simulink model "tx2"  (R2022a)
settings: Solver=FixedStepDiscrete  StartTime=0.0  StopTime=3.1e6  FixedStep=1  RelTol=1e-3
undefined symbols (not defined in the file or in its folder): rom_bf1, rom_bf2, rom_bf3, rom_bf4, rom_bf5, rom_bf6, rom_bf7, rom_bf8, rom_pilot_tt
libraries: hdlsllib x809, whdlutilities x460, whdlmod x104, whdledac x26, simulink x3
(part 8 of 27)

== system tx2/Subsystem6/mapping_process_L1 ==
  data_in : Inport  OutDataTypeStr=boolean
  mapping_ctrl : Inport  Port=2  OutDataTypeStr=Bus: samplecontrol
  Constant : Constant  Value=sqrt(2)/2  OutDataTypeStr=fixdt(1,16,14)
  Constant1 : Constant  Value=-sqrt(2)/2  OutDataTypeStr=fixdt(1,16,14)
  Constant2 : Constant  Value=0  OutDataTypeStr=uint8
  Constant3 : Constant  Value=0  OutDataTypeStr=fixdt(1,16,14)
  Delay : Delay  DelayLength=1  InitialCondition=0  ShowEnablePort=on
      settings: InputPortMap=u0,e6
  Delay{1,5..8,10..12} (8 alike) : Delay  DelayLength=1  InitialCondition=0
  Delay{3..4,9,13} (4 alike) : Delay  InitialCondition=0
  Delay2 : Delay  DelayLength=1  InitialCondition=0  ShowEnablePort=on
      settings: InputPortMap=u0,e6
  Demux : Demux  Outputs=2
  Logical Operator : Logic  Operator=OR  AllPortsSameDT=off  OutDataTypeStr=boolean
  Logical Operator1 : Logic  AllPortsSameDT=off  OutDataTypeStr=boolean
  Logical Operator13 : Logic  Operator=NOT  AllPortsSameDT=off  OutDataTypeStr=boolean
  Real-Imag to Complex : RealImagToComplex
  Real-Imag to Complex1 : RealImagToComplex
  Sample Control Bus Creator : whdlutilities/Sample Control Bus Creator
      settings: SourceProductBaseCode=LH
  Sample Control Bus Creator1 : whdlutilities/Sample Control Bus Creator
      settings: SourceProductBaseCode=LH
  Sample Control Bus Selector : whdlutilities/Sample Control Bus Selector  OutputSignals=start,end,valid
      settings: SourceProductBaseCode=LH
  Switch{,1..3} (4 alike) : Switch  Criteria=u2 ~= 0  SaturateOnIntegerOverflow=off  InputSameDT=off
  "divide6 " : hdlsllib/Sources/HDL Counter  CountType=Count limited  CountInit=1  CountStep=1  CountMax=12  CountFromType=Initial value  CountFrom=1  CountResetPort=on  CountLoadPort=off  CountEnbPort=on  CountDirPort=off  CountHitOutputPort=on  CountDataType=Unsigned  CountWordLen=8  CountFracLen=0  CountSampTime=1
  divide6 1 : hdlsllib/Sources/HDL Counter  CountType=Count limited  CountInit=1  CountStep=1  CountMax=6*12  CountFromType=Initial value  CountFrom=1  CountResetPort=on  CountLoadPort=off  CountEnbPort=on  CountDirPort=off  CountHitOutputPort=off  CountDataType=Unsigned  CountWordLen=8  CountFracLen=0  CountSampTime=1
  data_out : Outport  VectorParamsAs1DForOutWhenUnconnected=off
      settings: SignalType=complex
  ctrl_mapping : Outport  Port=2  OutDataTypeStr=Bus: samplecontrol  VectorParamsAs1DForOutWhenUnconnected=off
  RB_ctrl : Outport  Port=3  OutDataTypeStr=Bus: samplecontrol  VectorParamsAs1DForOutWhenUnconnected=off
  RB_id : Outport  Port=4  OutDataTypeStr=uint8  VectorParamsAs1DForOutWhenUnconnected=off
  wires:
  Switch1/1 -> Real-Imag to Complex/2
  Switch/1 -> Real-Imag to Complex/1
  Delay/1 -> Demux/1
  Demux/1 -> Switch/2
  Demux/2 -> Switch1/2
  Real-Imag to Complex/1 -> Delay2/1
  Delay2/1 -> Delay6/1
  Delay3/1 -> Delay5/1
  Delay1/1 -> Delay2/2, Delay13/1
  mapping_ctrl/1 -> Sample Control Bus Selector/1
  "divide6 "/2 -> divide6 1/2, Delay11/1, Delay10/1  "count6"
  Logical Operator13/1 -> divide6 1/1, "divide6 "/1
  Sample Control Bus Selector/1 -> Delay9/1, Sample Control Bus Creator/1  "<start>"
  Sample Control Bus Selector/2 -> Sample Control Bus Creator/2  "<end>"
  Sample Control Bus Selector/3 -> Sample Control Bus Creator/3, Delay4/1, Delay1/1, Delay/2  "<valid>"
  Sample Control Bus Creator/1 -> Delay3/1
  divide6 1/1 -> Switch2/1  "RB_id"
  Delay4/1 -> Logical Operator13/1, "divide6 "/2, Delay12/1, Switch2/2, Logical Operator1/1
  Switch2/1 -> Delay7/1
  Constant2/1 -> Switch2/3
  Delay6/1 -> Switch3/1
  Logical Operator/1 -> Logical Operator1/2
  Delay9/1 -> Logical Operator/2
  Delay10/1 -> Logical Operator/1
  Logical Operator1/1 -> Delay8/1
  Delay8/1 -> Sample Control Bus Creator1/1
  Delay11/1 -> Sample Control Bus Creator1/2
  Delay12/1 -> Sample Control Bus Creator1/3
  Delay5/1 -> ctrl_mapping/1
  Delay7/1 -> RB_id/1
  Sample Control Bus Creator1/1 -> RB_ctrl/1
  data_in/1 -> Delay/1  "data_with_CP"
  Switch3/1 -> data_out/1
  Constant3/1 -> Real-Imag to Complex1/2, Real-Imag to Complex1/1
  Real-Imag to Complex1/1 -> Switch3/3
  Delay13/1 -> Switch3/2
  Constant/1 -> Switch1/3, Switch/3
  Constant1/1 -> Switch/1, Switch1/1

== system tx2/Subsystem7/BF ==
  layer_data_in1 : Inport
  BF_data_ctrl : Inport  Port=2  OutDataTypeStr=Bus: samplecontrol
  RB_id : Inport  Port=3  OutDataTypeStr=uint8
  RB_id_ctrl : Inport  Port=4  OutDataTypeStr=Bus: samplecontrol
  Delay{,3..8,10} (8 alike) : Delay  DelayLength=1  InitialCondition=0
  Delay1 : Delay  InitialCondition=0
  Delay2 : Delay  DelayLength=3  InitialCondition=0
  Delay9 : Delay  InitialCondition=0
  Logical Operator : Logic  Operator=NOT  AllPortsSameDT=off  OutDataTypeStr=boolean
  Mux : Mux  Inputs=8
  Product{,1..7} (8 alike) : Product  OutDataTypeStr=fixdt(1,16,14)  LockScale=on
  Sample Control Bus Selector : whdlutilities/Sample Control Bus Selector  OutputSignals=start,end,valid
      settings: SourceProductBaseCode=LH
  Sample Control Bus Selector1 : whdlutilities/Sample Control Bus Selector  OutputSignals=start,end,valid
      settings: SourceProductBaseCode=LH
  address controller : hdlsllib/Sources/HDL Counter  CountType=Count limited  CountInit=0  CountStep=1  CountMax=7  CountFromType=Initial value  CountFrom=0  CountResetPort=on  CountLoadPort=off  CountEnbPort=on  CountDirPort=off  CountHitOutputPort=off  CountDataType=Unsigned  CountWordLen=8  CountFracLen=0  CountSampTime=1
  rom_bf1 : Subsystem
  rom_bf2 : Subsystem
  rom_bf3 : Subsystem
  rom_bf4 : Subsystem
  rom_bf5 : Subsystem
  rom_bf6 : Subsystem
  rom_bf7 : Subsystem
  rom_bf8 : Subsystem
  process_bf : Outport  PortDimensions=8  VectorParamsAs1DForOutWhenUnconnected=off
  BF_ctrl : Outport  Port=2  OutDataTypeStr=Bus: samplecontrol  VectorParamsAs1DForOutWhenUnconnected=off
  RB_n_bf : Outport  Port=3  VectorParamsAs1DForOutWhenUnconnected=off
  wires:
  Delay1/1 -> Product7/1, Product6/1, Product5/1, Product4/1, Product3/1, Product2/1, Product1/1, Product/1
  rom_bf1/1(data_out) -> Product/2
  Product/1 -> Delay/1
  Delay2/1 -> BF_ctrl/1  "BF_ctrl"
  address controller/1 -> rom_bf7/1(address), rom_bf8/1(address), rom_bf6/1(address), rom_bf5/1(address), rom_bf4/1(address), rom_bf3/1(address), rom_bf2/1(address), rom_bf1/1(address)
  Delay9/1 -> RB_n_bf/1  "RB_ID"
  RB_id_ctrl/1 -> Sample Control Bus Selector1/1
  BF_data_ctrl/1 -> Delay2/1, Sample Control Bus Selector/1
  Sample Control Bus Selector1/2 -> address controller/2  "<end>"
  RB_id/1 -> Delay9/1
  layer_data_in1/1 -> Delay1/1
  Sample Control Bus Selector/3 -> rom_bf2/2(read_en), rom_bf1/2(read_en), rom_bf3/2(read_en), rom_bf4/2(read_en), rom_bf5/2(read_en), rom_bf6/2(read_en), rom_bf7/2(read_en), rom_bf8/2(read_en)  "<valid>"
  Product1/1 -> Delay3/1
  Product2/1 -> Delay4/1
  Product4/1 -> Delay6/1
  Product3/1 -> Delay5/1
  Product5/1 -> Delay7/1
  Product6/1 -> Delay8/1
  rom_bf2/1(data_out) -> Product1/2
  rom_bf3/1(data_out) -> Product2/2
  rom_bf4/1(data_out) -> Product3/2
  rom_bf5/1(data_out) -> Product4/2
  rom_bf6/1(data_out) -> Product5/2
  Product7/1 -> Delay10/1
  rom_bf7/1(data_out) -> Product6/2
  rom_bf8/1(data_out) -> Product7/2
  Delay3/1 -> Mux/2
  Delay4/1 -> Mux/3
  Delay5/1 -> Mux/4
  Delay10/1 -> Mux/8
  Delay8/1 -> Mux/7
  Delay7/1 -> Mux/6
  Delay6/1 -> Mux/5
  Delay/1 -> Mux/1
  Mux/1 -> process_bf/1
  Sample Control Bus Selector1/3 -> Logical Operator/1  "<valid>"
  Logical Operator/1 -> address controller/1

== system tx2/Subsystem7/OFDM_process1 ==
  process_bf : Inport
  BF_ctrl : Inport  Port=2
  Demux : Demux  Outputs=8
  OFDM_process1_bf1 : Subsystem
  OFDM_process1_bf2 : Subsystem
  OFDM_process1_bf3 : Subsystem
  OFDM_process1_bf4 : Subsystem
  OFDM_process1_bf5 : Subsystem
  OFDM_process1_bf6 : Subsystem
  OFDM_process1_bf7 : Subsystem
  OFDM_process1_bf8 : Subsystem
  OFDM_bf1 : Outport
  OFDM_ctrl_bf1 : Outport  Port=2
  OFDM_bf2 : Outport  Port=3
  OFDM_ctrl_bf2 : Outport  Port=4
  OFDM_bf3 : Outport  Port=5
  OFDM_ctrl_bf3 : Outport  Port=6
  OFDM_bf4 : Outport  Port=7
  OFDM_ctrl_bf4 : Outport  Port=8
  OFDM_bf5 : Outport  Port=9
  OFDM_ctrl_bf5 : Outport  Port=10
  OFDM_bf6 : Outport  Port=11
  OFDM_ctrl_bf6 : Outport  Port=12
  OFDM_bf7 : Outport  Port=13
  OFDM_ctrl_bf7 : Outport  Port=14
  OFDM_bf8 : Outport  Port=15
  OFDM_ctrl_bf8 : Outport  Port=16
  wires:
  Demux/3 -> OFDM_process1_bf3/1(data)  "bf3"
  Demux/1 -> OFDM_process1_bf1/1(data)  "bf1"
  BF_ctrl/1 -> OFDM_process1_bf7/2(BF_ctrl), OFDM_process1_bf8/2(BF_ctrl), OFDM_process1_bf6/2(BF_ctrl), OFDM_process1_bf5/2(BF_ctrl), OFDM_process1_bf4/2(BF_ctrl), OFDM_process1_bf3/2(BF_ctrl), OFDM_process1_bf2/2(BF_ctrl), OFDM_process1_bf1/2(BF_ctrl)
  Demux/5 -> OFDM_process1_bf5/1(data)  "bf5"
  OFDM_process1_bf1/2(OFDM_ctrl_process) -> OFDM_ctrl_bf1/1
  OFDM_process1_bf2/2(OFDM_ctrl_process) -> OFDM_ctrl_bf2/1
  Demux/2 -> OFDM_process1_bf2/1(data)  "bf2"
  Demux/4 -> OFDM_process1_bf4/1(data)  "bf4"
  OFDM_process1_bf8/2(OFDM_ctrl_process) -> OFDM_ctrl_bf8/1
  Demux/8 -> OFDM_process1_bf8/1(data)  "bf8"
  Demux/7 -> OFDM_process1_bf7/1(data)  "bf7"
  Demux/6 -> OFDM_process1_bf6/1(data)  "bf6"
  OFDM_process1_bf7/2(OFDM_ctrl_process) -> OFDM_ctrl_bf7/1
  OFDM_process1_bf6/1(OFDM_process) -> OFDM_bf6/1
  OFDM_process1_bf3/1(OFDM_process) -> OFDM_bf3/1
  OFDM_process1_bf6/2(OFDM_ctrl_process) -> OFDM_ctrl_bf6/1
  OFDM_process1_bf5/1(OFDM_process) -> OFDM_bf5/1
  OFDM_process1_bf1/1(OFDM_process) -> OFDM_bf1/1
  OFDM_process1_bf8/1(OFDM_process) -> OFDM_bf8/1
  OFDM_process1_bf4/2(OFDM_ctrl_process) -> OFDM_ctrl_bf4/1
  OFDM_process1_bf3/2(OFDM_ctrl_process) -> OFDM_ctrl_bf3/1
  OFDM_process1_bf5/2(OFDM_ctrl_process) -> OFDM_ctrl_bf5/1
  process_bf/1 -> Demux/1
  OFDM_process1_bf7/1(OFDM_process) -> OFDM_bf7/1
  OFDM_process1_bf4/1(OFDM_process) -> OFDM_bf4/1
  OFDM_process1_bf2/1(OFDM_process) -> OFDM_bf2/1

== system tx2/Subsystem7/bit_level ==
  note: 此时的输出本身具有一位延迟
  process_data : Inport
  process_valid : Inport  Port=2  OutDataTypeStr=Bus: samplecontrol
  Compare To Constant1 : hdlsllib/Logic and Bit Operations/Compare To Constant  relop=<  const=385  OutDataTypeStr=boolean
      settings: SourceProductBaseCode=SL
  Compare To Constant2 : hdlsllib/Logic and Bit Operations/Compare To Constant  relop===  const=1584+192  OutDataTypeStr=boolean
      settings: SourceProductBaseCode=SL
  Compare To Constant3 : hdlsllib/Logic and Bit Operations/Compare To Constant  relop=>  const=576  OutDataTypeStr=boolean
      settings: SourceProductBaseCode=SL
  Compare To Constant4 : hdlsllib/Logic and Bit Operations/Compare To Constant  relop=<=  const=1584+192  OutDataTypeStr=boolean
      settings: SourceProductBaseCode=SL
  Compare To Constant5 : hdlsllib/Logic and Bit Operations/Compare To Constant  relop=>=  const=792+1  OutDataTypeStr=boolean
      settings: SourceProductBaseCode=SL
  Compare To Constant6 : hdlsllib/Logic and Bit Operations/Compare To Constant  relop=<=  const=1584  OutDataTypeStr=boolean
      settings: SourceProductBaseCode=SL
  Constant : Constant  OutDataTypeStr=boolean
  Constant1 : Constant  Value=72  OutDataTypeStr=uint16
  Constant2 : Constant  Value=0  OutDataTypeStr=boolean
  Constant3 : Constant  Value=0  OutDataTypeStr=fixdt(0,12,0)
  Data Type Conversion1 : DataTypeConversion  OutDataTypeStr=fixdt(0,1,0)  SaturateOnIntegerOverflow=off  RndMeth=Floor
  Data Type Conversion2 : DataTypeConversion  OutDataTypeStr=boolean  SaturateOnIntegerOverflow=off  RndMeth=Floor
  Data Type Conversion3 : DataTypeConversion  OutDataTypeStr=boolean  SaturateOnIntegerOverflow=off  RndMeth=Floor
  Delay1 : Delay  DelayLength=1  InitialCondition=0
  Delay2 : Delay  DelayLength=1  InitialCondition=0
  HDL Counter1 : hdlsllib/Sources/HDL Counter  CountType=Count limited  CountInit=1  CountStep=1  CountMax=1584  CountFromType=Initial value  CountFrom=1  CountResetPort=on  CountLoadPort=off  CountEnbPort=on  CountDirPort=off  CountHitOutputPort=off  CountDataType=Unsigned  CountWordLen=12  CountFracLen=0  CountSampTime=1
  HDL Counter2 : hdlsllib/Sources/HDL Counter  CountType=Count limited  CountInit=1  CountStep=1  CountMax=792  CountFromType=Initial value  CountFrom=1  CountResetPort=on  CountLoadPort=off  CountEnbPort=on  CountDirPort=off  CountHitOutputPort=off  CountDataType=Unsigned  CountWordLen=12  CountFracLen=0  CountSampTime=1
  HDL Counter4 : hdlsllib/Sources/HDL Counter  CountType=Count limited  CountInit=1  CountStep=1  CountMax=4096-1  CountFromType=Initial value  CountFrom=1  CountResetPort=on  CountLoadPort=off  CountEnbPort=on  CountDirPort=off  CountHitOutputPort=off  CountDataType=Unsigned  CountWordLen=12  CountFracLen=0  CountSampTime=1
  HDL Counter5 : hdlsllib/Sources/HDL Counter  CountType=Count limited  CountInit=0  CountStep=1  CountMax=1  CountFromType=Initial value  CountFrom=0  CountResetPort=on  CountLoadPort=off  CountEnbPort=on  CountDirPort=off  CountHitOutputPort=off  CountDataType=Unsigned  CountWordLen=1  CountFracLen=0  CountSampTime=1
  Logical Operator : Logic  Operator=OR  AllPortsSameDT=off  OutDataTypeStr=boolean
  Logical Operator{1,3,7..8} (4 alike) : Logic  Operator=NOT  AllPortsSameDT=off  OutDataTypeStr=boolean
  Logical Operator{2,4..6} (4 alike) : Logic  AllPortsSameDT=off  OutDataTypeStr=boolean
  Mux : Mux  Inputs=2
  NR CRC Encoder : whdledac/NR CRC Encoder  CRCType=CRC16  EnableCRCMaskPort=off  SimulateUsing=Code generation
      settings: SourceProductBaseCode=LH
  NR LDPC Encoder2 : whdledac/NR LDPC Encoder
      settings: SourceProductBaseCode=LH
  Sample Control Bus Creator : whdlutilities/Sample Control Bus Creator
      settings: SourceProductBaseCode=LH
  Sample Control Bus Selector : whdlutilities/Sample Control Bus Selector  OutputSignals=start,end,valid
      settings: SourceProductBaseCode=LH
  Sample Control Bus Selector1 : whdlutilities/Sample Control Bus Selector  OutputSignals=start,end,valid
      settings: SourceProductBaseCode=LH
  Simple Dual Port RAM1 : hdlsllib/HDL RAMs/Simple Dual Port RAM  ram_size=12
      settings: SourceProductBaseCode=SL
  Subsystem : Subsystem
  Switch : Switch  Criteria=u2 ~= 0  SaturateOnIntegerOverflow=off  InputSameDT=off
  Switch1 : Switch  Criteria=u2 ~= 0  SaturateOnIntegerOverflow=off  InputSameDT=off
  Switch2 : Switch  Criteria=u2 ~= 0  SaturateOnIntegerOverflow=off  InputSameDT=off
  ctrl_gen : Subsystem
  valid_recover : Subsystem
  bit_level_process : Outport  OutDataTypeStr=boolean
  "bit_level_ctrl_process " : Outport  Port=2  OutDataTypeStr=Bus: samplecontrol
  wires:
  ctrl_gen/1(data_out) -> bit_level_process/1  "INTERLEAVE"
  process_valid/1 -> NR CRC Encoder/2
  Delay2/1 -> ctrl_gen/2(select_valid)
  Delay1/1 -> Mux/2
  Compare To Constant4/1 -> Logical Operator2/2
  Mux/1 -> ctrl_gen/1(data_in)
  Sample Control Bus Creator/1 -> NR LDPC Encoder2/2
  NR CRC Encoder/2 -> Sample Control Bus Selector/1
  Compare To Constant1/1 -> Logical Operator/1
  Compare To Constant2/1 -> HDL Counter5/2
  Constant2/1 -> Switch/3
  Compare To Constant6/1 -> Logical Operator6/2
  HDL Counter4/1 -> Compare To Constant2/1, Compare To Constant3/1, Compare To Constant4/1, Compare To Constant1/1  "wr_addr"
  Data Type Conversion1/1 -> Simple Dual Port RAM1/1  "wr_din"
  Compare To Constant5/1 -> Logical Operator6/1
  Logical Operator5/1 -> Simple Dual Port RAM1/3, Switch1/2, HDL Counter1/2  "wr_en"
  Compare To Constant3/1 -> Logical Operator/2
  Subsystem/1(end_out) -> valid_recover/3(end_in)
  process_data/1 -> NR CRC Encoder/1
  Data Type Conversion2/1 -> HDL Counter4/1
  Switch1/1 -> Simple Dual Port RAM1/2  "wr_addr"
  Logical Operator6/1 -> Switch/2, Delay2/1, Logical Operator7/1, Switch2/2, HDL Counter2/2
  Logical Operator1/1 -> HDL Counter1/1
  valid_recover/1(data_out) -> NR LDPC Encoder2/1
  NR LDPC Encoder2/2 -> Sample Control Bus Selector1/1
  HDL Counter1/1 -> Compare To Constant5/1, Compare To Constant6/1, Switch1/1
  Switch2/1 -> Simple Dual Port RAM1/4  "rd_addr"
  valid_recover/4(valid_out) -> Sample Control Bus Creator/3
  Logical Operator/1 -> Logical Operator2/1
  Logical Operator4/1 -> Logical Operator5/2
  Logical Operator3/1 -> Logical Operator4/1
  Logical Operator7/1 -> HDL Counter2/1
  Logical Operator2/1 -> Logical Operator5/1
  Sample Control Bus Selector1/3 -> Logical Operator4/2, Logical Operator1/1, Logical Operator8/1, HDL Counter4/2  "<valid>"
  valid_recover/3(end_out) -> Sample Control Bus Creator/2
  valid_recover/2(start_out) -> Sample Control Bus Creator/1
  Sample Control Bus Selector/1 -> valid_recover/2(start_in)  "<start>"
  Simple Dual Port RAM1/1 -> Data Type Conversion3/1
  NR LDPC Encoder2/1 -> Data Type Conversion1/1, Switch/1  "LDPC"
  Sample Control Bus Selector/2 -> Subsystem/1(end_in)  "<end>"
  Logical Operator8/1 -> HDL Counter5/1
  HDL Counter2/1 -> Switch2/1  "rd_addr"
  Constant1/1 -> NR LDPC Encoder2/4
  ctrl_gen/2(ctrl_out) -> "bit_level_ctrl_process "/1
  NR CRC Encoder/1 -> valid_recover/1(data_in)  "CRC"
  Constant3/1 -> Switch1/3, Switch2/3
  Constant/1 -> NR LDPC Encoder2/3
  Data Type Conversion3/1 -> Mux/1
  HDL Counter5/1 -> Data Type Conversion2/1, Logical Operator3/1  "loop_ctrl"
  Switch/1 -> Delay1/1

== system tx2/Subsystem7/mapping_process_L1 ==
  data_in : Inport  OutDataTypeStr=boolean
  mapping_ctrl : Inport  Port=2  OutDataTypeStr=Bus: samplecontrol
  Constant : Constant  Value=sqrt(2)/2  OutDataTypeStr=fixdt(1,16,14)
  Constant1 : Constant  Value=-sqrt(2)/2  OutDataTypeStr=fixdt(1,16,14)
  Constant2 : Constant  Value=0  OutDataTypeStr=uint8
  Constant3 : Constant  Value=0  OutDataTypeStr=fixdt(1,16,14)
  Delay : Delay  DelayLength=1  InitialCondition=0  ShowEnablePort=on
      settings: InputPortMap=u0,e6
  Delay{1,5..8,10..12} (8 alike) : Delay  DelayLength=1  InitialCondition=0
  Delay{3..4,9,13} (4 alike) : Delay  InitialCondition=0
  Delay2 : Delay  DelayLength=1  InitialCondition=0  ShowEnablePort=on
      settings: InputPortMap=u0,e6
  Demux : Demux  Outputs=2
  Logical Operator : Logic  Operator=OR  AllPortsSameDT=off  OutDataTypeStr=boolean
  Logical Operator1 : Logic  AllPortsSameDT=off  OutDataTypeStr=boolean
  Logical Operator13 : Logic  Operator=NOT  AllPortsSameDT=off  OutDataTypeStr=boolean
  Real-Imag to Complex : RealImagToComplex
  Real-Imag to Complex1 : RealImagToComplex
  Sample Control Bus Creator : whdlutilities/Sample Control Bus Creator
      settings: SourceProductBaseCode=LH
  Sample Control Bus Creator1 : whdlutilities/Sample Control Bus Creator
      settings: SourceProductBaseCode=LH
  Sample Control Bus Selector : whdlutilities/Sample Control Bus Selector  OutputSignals=start,end,valid
      settings: SourceProductBaseCode=LH
  Switch{,1..3} (4 alike) : Switch  Criteria=u2 ~= 0  SaturateOnIntegerOverflow=off  InputSameDT=off
  "divide6 " : hdlsllib/Sources/HDL Counter  CountType=Count limited  CountInit=1  CountStep=1  CountMax=12  CountFromType=Initial value  CountFrom=1  CountResetPort=on  CountLoadPort=off  CountEnbPort=on  CountDirPort=off  CountHitOutputPort=on  CountDataType=Unsigned  CountWordLen=8  CountFracLen=0  CountSampTime=1
  divide6 1 : hdlsllib/Sources/HDL Counter  CountType=Count limited  CountInit=1  CountStep=1  CountMax=6*12  CountFromType=Initial value  CountFrom=1  CountResetPort=on  CountLoadPort=off  CountEnbPort=on  CountDirPort=off  CountHitOutputPort=off  CountDataType=Unsigned  CountWordLen=8  CountFracLen=0  CountSampTime=1
  data_out : Outport  VectorParamsAs1DForOutWhenUnconnected=off
      settings: SignalType=complex
  ctrl_mapping : Outport  Port=2  OutDataTypeStr=Bus: samplecontrol  VectorParamsAs1DForOutWhenUnconnected=off
  RB_ctrl : Outport  Port=3  OutDataTypeStr=Bus: samplecontrol  VectorParamsAs1DForOutWhenUnconnected=off
  RB_id : Outport  Port=4  OutDataTypeStr=uint8  VectorParamsAs1DForOutWhenUnconnected=off
  wires:
  Constant1/1 -> Switch1/1, Switch/1
  Constant/1 -> Switch/3, Switch1/3
  Delay13/1 -> Switch3/2
  Real-Imag to Complex1/1 -> Switch3/3
  Constant3/1 -> Real-Imag to Complex1/1, Real-Imag to Complex1/2
  Switch3/1 -> data_out/1
  data_in/1 -> Delay/1  "data_with_CP"
  Sample Control Bus Creator1/1 -> RB_ctrl/1
  Delay7/1 -> RB_id/1
  Delay5/1 -> ctrl_mapping/1
  Delay12/1 -> Sample Control Bus Creator1/3
  Delay11/1 -> Sample Control Bus Creator1/2
  Delay8/1 -> Sample Control Bus Creator1/1
  Logical Operator1/1 -> Delay8/1
  Delay10/1 -> Logical Operator/1
  Delay9/1 -> Logical Operator/2
  Logical Operator/1 -> Logical Operator1/2
  Delay6/1 -> Switch3/1
  Constant2/1 -> Switch2/3
  Switch2/1 -> Delay7/1
  Delay4/1 -> Logical Operator1/1, Switch2/2, Delay12/1, "divide6 "/2, Logical Operator13/1
  divide6 1/1 -> Switch2/1  "RB_id"
  Sample Control Bus Creator/1 -> Delay3/1
  Sample Control Bus Selector/3 -> Delay/2, Delay1/1, Delay4/1, Sample Control Bus Creator/3  "<valid>"
  Sample Control Bus Selector/2 -> Sample Control Bus Creator/2  "<end>"
  Sample Control Bus Selector/1 -> Sample Control Bus Creator/1, Delay9/1  "<start>"
  Logical Operator13/1 -> "divide6 "/1, divide6 1/1
  "divide6 "/2 -> Delay10/1, Delay11/1, divide6 1/2  "count6"
  mapping_ctrl/1 -> Sample Control Bus Selector/1
  Delay1/1 -> Delay13/1, Delay2/2
  Delay3/1 -> Delay5/1
  Delay2/1 -> Delay6/1
  Real-Imag to Complex/1 -> Delay2/1
  Demux/2 -> Switch1/2
  Demux/1 -> Switch/2
  Delay/1 -> Demux/1
  Switch/1 -> Real-Imag to Complex/1
  Switch1/1 -> Real-Imag to Complex/2

== system tx2/Subsystem8/BF ==
  layer_data_in1 : Inport
  BF_data_ctrl : Inport  Port=2  OutDataTypeStr=Bus: samplecontrol
  RB_id : Inport  Port=3  OutDataTypeStr=uint8
  RB_id_ctrl : Inport  Port=4  OutDataTypeStr=Bus: samplecontrol
  Delay{,3..8,10} (8 alike) : Delay  DelayLength=1  InitialCondition=0
  Delay1 : Delay  InitialCondition=0
  Delay2 : Delay  DelayLength=3  InitialCondition=0
  Delay9 : Delay  InitialCondition=0
  Logical Operator : Logic  Operator=NOT  AllPortsSameDT=off  OutDataTypeStr=boolean
  Mux : Mux  Inputs=8
  Product{,1..7} (8 alike) : Product  OutDataTypeStr=fixdt(1,16,14)  LockScale=on
  Sample Control Bus Selector : whdlutilities/Sample Control Bus Selector  OutputSignals=start,end,valid
      settings: SourceProductBaseCode=LH
  Sample Control Bus Selector1 : whdlutilities/Sample Control Bus Selector  OutputSignals=start,end,valid
      settings: SourceProductBaseCode=LH
  address controller : hdlsllib/Sources/HDL Counter  CountType=Count limited  CountInit=0  CountStep=1  CountMax=7  CountFromType=Initial value  CountFrom=0  CountResetPort=on  CountLoadPort=off  CountEnbPort=on  CountDirPort=off  CountHitOutputPort=off  CountDataType=Unsigned  CountWordLen=8  CountFracLen=0  CountSampTime=1
  rom_bf1 : Subsystem
  rom_bf2 : Subsystem
  rom_bf3 : Subsystem
  rom_bf4 : Subsystem
  rom_bf5 : Subsystem
  rom_bf6 : Subsystem
  rom_bf7 : Subsystem
  rom_bf8 : Subsystem
  process_bf : Outport  PortDimensions=8  VectorParamsAs1DForOutWhenUnconnected=off
  BF_ctrl : Outport  Port=2  OutDataTypeStr=Bus: samplecontrol  VectorParamsAs1DForOutWhenUnconnected=off
  RB_n_bf : Outport  Port=3  VectorParamsAs1DForOutWhenUnconnected=off
  wires:
  Delay1/1 -> Product7/1, Product6/1, Product5/1, Product4/1, Product3/1, Product2/1, Product1/1, Product/1
  rom_bf1/1(data_out) -> Product/2
  Product/1 -> Delay/1
  Delay2/1 -> BF_ctrl/1  "BF_ctrl"
  address controller/1 -> rom_bf7/1(address), rom_bf8/1(address), rom_bf6/1(address), rom_bf5/1(address), rom_bf4/1(address), rom_bf3/1(address), rom_bf2/1(address), rom_bf1/1(address)
  Delay9/1 -> RB_n_bf/1  "RB_ID"
  RB_id_ctrl/1 -> Sample Control Bus Selector1/1
  BF_data_ctrl/1 -> Delay2/1, Sample Control Bus Selector/1
  Sample Control Bus Selector1/2 -> address controller/2  "<end>"
  RB_id/1 -> Delay9/1
  layer_data_in1/1 -> Delay1/1
  Sample Control Bus Selector/3 -> rom_bf2/2(read_en), rom_bf1/2(read_en), rom_bf3/2(read_en), rom_bf4/2(read_en), rom_bf5/2(read_en), rom_bf6/2(read_en), rom_bf7/2(read_en), rom_bf8/2(read_en)  "<valid>"
  Product1/1 -> Delay3/1
  Product2/1 -> Delay4/1
  Product4/1 -> Delay6/1
  Product3/1 -> Delay5/1
  Product5/1 -> Delay7/1
  Product6/1 -> Delay8/1
  rom_bf2/1(data_out) -> Product1/2
  rom_bf3/1(data_out) -> Product2/2
  rom_bf4/1(data_out) -> Product3/2
  rom_bf5/1(data_out) -> Product4/2
  rom_bf6/1(data_out) -> Product5/2
  Product7/1 -> Delay10/1
  rom_bf7/1(data_out) -> Product6/2
  rom_bf8/1(data_out) -> Product7/2
  Delay3/1 -> Mux/2
  Delay4/1 -> Mux/3
  Delay5/1 -> Mux/4
  Delay10/1 -> Mux/8
  Delay8/1 -> Mux/7
  Delay7/1 -> Mux/6
  Delay6/1 -> Mux/5
  Delay/1 -> Mux/1
  Mux/1 -> process_bf/1
  Sample Control Bus Selector1/3 -> Logical Operator/1  "<valid>"
  Logical Operator/1 -> address controller/1

== system tx2/Subsystem8/OFDM_process1 ==
  process_bf : Inport
  BF_ctrl : Inport  Port=2
  Demux : Demux  Outputs=8
  OFDM_process1_bf1 : Subsystem
  OFDM_process1_bf2 : Subsystem
  OFDM_process1_bf3 : Subsystem
  OFDM_process1_bf4 : Subsystem
  OFDM_process1_bf5 : Subsystem
  OFDM_process1_bf6 : Subsystem
  OFDM_process1_bf7 : Subsystem
  OFDM_process1_bf8 : Subsystem
  OFDM_bf1 : Outport
  OFDM_ctrl_bf1 : Outport  Port=2
  OFDM_bf2 : Outport  Port=3
  OFDM_ctrl_bf2 : Outport  Port=4
  OFDM_bf3 : Outport  Port=5
  OFDM_ctrl_bf3 : Outport  Port=6
  OFDM_bf4 : Outport  Port=7
  OFDM_ctrl_bf4 : Outport  Port=8
  OFDM_bf5 : Outport  Port=9
  OFDM_ctrl_bf5 : Outport  Port=10
  OFDM_bf6 : Outport  Port=11
  OFDM_ctrl_bf6 : Outport  Port=12
  OFDM_bf7 : Outport  Port=13
  OFDM_ctrl_bf7 : Outport  Port=14
  OFDM_bf8 : Outport  Port=15
  OFDM_ctrl_bf8 : Outport  Port=16
  wires:
  OFDM_process1_bf2/1(OFDM_process) -> OFDM_bf2/1
  OFDM_process1_bf4/1(OFDM_process) -> OFDM_bf4/1
  OFDM_process1_bf7/1(OFDM_process) -> OFDM_bf7/1
  process_bf/1 -> Demux/1
  OFDM_process1_bf5/2(OFDM_ctrl_process) -> OFDM_ctrl_bf5/1
  OFDM_process1_bf3/2(OFDM_ctrl_process) -> OFDM_ctrl_bf3/1
  OFDM_process1_bf4/2(OFDM_ctrl_process) -> OFDM_ctrl_bf4/1
  OFDM_process1_bf8/1(OFDM_process) -> OFDM_bf8/1
  OFDM_process1_bf1/1(OFDM_process) -> OFDM_bf1/1
  OFDM_process1_bf5/1(OFDM_process) -> OFDM_bf5/1
  OFDM_process1_bf6/2(OFDM_ctrl_process) -> OFDM_ctrl_bf6/1
  OFDM_process1_bf3/1(OFDM_process) -> OFDM_bf3/1
  OFDM_process1_bf6/1(OFDM_process) -> OFDM_bf6/1
  OFDM_process1_bf7/2(OFDM_ctrl_process) -> OFDM_ctrl_bf7/1
  Demux/6 -> OFDM_process1_bf6/1(data)  "bf6"
  Demux/7 -> OFDM_process1_bf7/1(data)  "bf7"
  Demux/8 -> OFDM_process1_bf8/1(data)  "bf8"
  OFDM_process1_bf8/2(OFDM_ctrl_process) -> OFDM_ctrl_bf8/1
  Demux/4 -> OFDM_process1_bf4/1(data)  "bf4"
  Demux/2 -> OFDM_process1_bf2/1(data)  "bf2"
  OFDM_process1_bf2/2(OFDM_ctrl_process) -> OFDM_ctrl_bf2/1
  OFDM_process1_bf1/2(OFDM_ctrl_process) -> OFDM_ctrl_bf1/1
  Demux/5 -> OFDM_process1_bf5/1(data)  "bf5"
  BF_ctrl/1 -> OFDM_process1_bf1/2(BF_ctrl), OFDM_process1_bf2/2(BF_ctrl), OFDM_process1_bf3/2(BF_ctrl), OFDM_process1_bf4/2(BF_ctrl), OFDM_process1_bf5/2(BF_ctrl), OFDM_process1_bf6/2(BF_ctrl), OFDM_process1_bf8/2(BF_ctrl), OFDM_process1_bf7/2(BF_ctrl)
  Demux/1 -> OFDM_process1_bf1/1(data)  "bf1"
  Demux/3 -> OFDM_process1_bf3/1(data)  "bf3"

== system tx2/Subsystem8/bit_level ==
  note: 此时的输出本身具有一位延迟
  process_data : Inport
  process_valid : Inport  Port=2  OutDataTypeStr=Bus: samplecontrol
  Compare To Constant1 : hdlsllib/Logic and Bit Operations/Compare To Constant  relop=<  const=385  OutDataTypeStr=boolean
      settings: SourceProductBaseCode=SL
  Compare To Constant2 : hdlsllib/Logic and Bit Operations/Compare To Constant  relop===  const=1584+192  OutDataTypeStr=boolean
      settings: SourceProductBaseCode=SL
  Compare To Constant3 : hdlsllib/Logic and Bit Operations/Compare To Constant  relop=>  const=576  OutDataTypeStr=boolean
      settings: SourceProductBaseCode=SL
  Compare To Constant4 : hdlsllib/Logic and Bit Operations/Compare To Constant  relop=<=  const=1584+192  OutDataTypeStr=boolean
      settings: SourceProductBaseCode=SL
  Compare To Constant5 : hdlsllib/Logic and Bit Operations/Compare To Constant  relop=>=  const=792+1  OutDataTypeStr=boolean
      settings: SourceProductBaseCode=SL
  Compare To Constant6 : hdlsllib/Logic and Bit Operations/Compare To Constant  relop=<=  const=1584  OutDataTypeStr=boolean
      settings: SourceProductBaseCode=SL
  Constant : Constant  OutDataTypeStr=boolean
  Constant1 : Constant  Value=72  OutDataTypeStr=uint16
  Constant2 : Constant  Value=0  OutDataTypeStr=boolean
  Constant3 : Constant  Value=0  OutDataTypeStr=fixdt(0,12,0)
  Data Type Conversion1 : DataTypeConversion  OutDataTypeStr=fixdt(0,1,0)  SaturateOnIntegerOverflow=off  RndMeth=Floor
  Data Type Conversion2 : DataTypeConversion  OutDataTypeStr=boolean  SaturateOnIntegerOverflow=off  RndMeth=Floor
  Data Type Conversion3 : DataTypeConversion  OutDataTypeStr=boolean  SaturateOnIntegerOverflow=off  RndMeth=Floor
  Delay1 : Delay  DelayLength=1  InitialCondition=0
  Delay2 : Delay  DelayLength=1  InitialCondition=0
  HDL Counter1 : hdlsllib/Sources/HDL Counter  CountType=Count limited  CountInit=1  CountStep=1  CountMax=1584  CountFromType=Initial value  CountFrom=1  CountResetPort=on  CountLoadPort=off  CountEnbPort=on  CountDirPort=off  CountHitOutputPort=off  CountDataType=Unsigned  CountWordLen=12  CountFracLen=0  CountSampTime=1
  HDL Counter2 : hdlsllib/Sources/HDL Counter  CountType=Count limited  CountInit=1  CountStep=1  CountMax=792  CountFromType=Initial value  CountFrom=1  CountResetPort=on  CountLoadPort=off  CountEnbPort=on  CountDirPort=off  CountHitOutputPort=off  CountDataType=Unsigned  CountWordLen=12  CountFracLen=0  CountSampTime=1
  HDL Counter4 : hdlsllib/Sources/HDL Counter  CountType=Count limited  CountInit=1  CountStep=1  CountMax=4096-1  CountFromType=Initial value  CountFrom=1  CountResetPort=on  CountLoadPort=off  CountEnbPort=on  CountDirPort=off  CountHitOutputPort=off  CountDataType=Unsigned  CountWordLen=12  CountFracLen=0  CountSampTime=1
  HDL Counter5 : hdlsllib/Sources/HDL Counter  CountType=Count limited  CountInit=0  CountStep=1  CountMax=1  CountFromType=Initial value  CountFrom=0  CountResetPort=on  CountLoadPort=off  CountEnbPort=on  CountDirPort=off  CountHitOutputPort=off  CountDataType=Unsigned  CountWordLen=1  CountFracLen=0  CountSampTime=1
  Logical Operator : Logic  Operator=OR  AllPortsSameDT=off  OutDataTypeStr=boolean
  Logical Operator{1,3,7..8} (4 alike) : Logic  Operator=NOT  AllPortsSameDT=off  OutDataTypeStr=boolean
  Logical Operator{2,4..6} (4 alike) : Logic  AllPortsSameDT=off  OutDataTypeStr=boolean
  Mux : Mux  Inputs=2
  NR CRC Encoder : whdledac/NR CRC Encoder  CRCType=CRC16  EnableCRCMaskPort=off  SimulateUsing=Code generation
      settings: SourceProductBaseCode=LH
  NR LDPC Encoder2 : whdledac/NR LDPC Encoder
      settings: SourceProductBaseCode=LH
  Sample Control Bus Creator : whdlutilities/Sample Control Bus Creator
      settings: SourceProductBaseCode=LH
  Sample Control Bus Selector : whdlutilities/Sample Control Bus Selector  OutputSignals=start,end,valid
      settings: SourceProductBaseCode=LH
  Sample Control Bus Selector1 : whdlutilities/Sample Control Bus Selector  OutputSignals=start,end,valid
      settings: SourceProductBaseCode=LH
  Simple Dual Port RAM1 : hdlsllib/HDL RAMs/Simple Dual Port RAM  ram_size=12
      settings: SourceProductBaseCode=SL
  Subsystem : Subsystem
  Switch : Switch  Criteria=u2 ~= 0  SaturateOnIntegerOverflow=off  InputSameDT=off
  Switch1 : Switch  Criteria=u2 ~= 0  SaturateOnIntegerOverflow=off  InputSameDT=off
  Switch2 : Switch  Criteria=u2 ~= 0  SaturateOnIntegerOverflow=off  InputSameDT=off
  ctrl_gen : Subsystem
  valid_recover : Subsystem
  bit_level_process : Outport  OutDataTypeStr=boolean
  "bit_level_ctrl_process " : Outport  Port=2  OutDataTypeStr=Bus: samplecontrol
  wires:
  Switch/1 -> Delay1/1
  HDL Counter5/1 -> Logical Operator3/1, Data Type Conversion2/1  "loop_ctrl"
  Data Type Conversion3/1 -> Mux/1
  Constant/1 -> NR LDPC Encoder2/3
  Constant3/1 -> Switch2/3, Switch1/3
  NR CRC Encoder/1 -> valid_recover/1(data_in)  "CRC"
  ctrl_gen/2(ctrl_out) -> "bit_level_ctrl_process "/1
  Constant1/1 -> NR LDPC Encoder2/4
  HDL Counter2/1 -> Switch2/1  "rd_addr"
  Logical Operator8/1 -> HDL Counter5/1
  Sample Control Bus Selector/2 -> Subsystem/1(end_in)  "<end>"
  NR LDPC Encoder2/1 -> Switch/1, Data Type Conversion1/1  "LDPC"
  Simple Dual Port RAM1/1 -> Data Type Conversion3/1
  Sample Control Bus Selector/1 -> valid_recover/2(start_in)  "<start>"
  valid_recover/2(start_out) -> Sample Control Bus Creator/1
  valid_recover/3(end_out) -> Sample Control Bus Creator/2
  Sample Control Bus Selector1/3 -> HDL Counter4/2, Logical Operator8/1, Logical Operator1/1, Logical Operator4/2  "<valid>"
  Logical Operator2/1 -> Logical Operator5/1
  Logical Operator7/1 -> HDL Counter2/1
  Logical Operator3/1 -> Logical Operator4/1
  Logical Operator4/1 -> Logical Operator5/2
  Logical Operator/1 -> Logical Operator2/1
  valid_recover/4(valid_out) -> Sample Control Bus Creator/3
  Switch2/1 -> Simple Dual Port RAM1/4  "rd_addr"
  HDL Counter1/1 -> Switch1/1, Compare To Constant6/1, Compare To Constant5/1
  NR LDPC Encoder2/2 -> Sample Control Bus Selector1/1
  valid_recover/1(data_out) -> NR LDPC Encoder2/1
  Logical Operator1/1 -> HDL Counter1/1
  Logical Operator6/1 -> HDL Counter2/2, Switch2/2, Logical Operator7/1, Delay2/1, Switch/2
  Switch1/1 -> Simple Dual Port RAM1/2  "wr_addr"
  Data Type Conversion2/1 -> HDL Counter4/1
  process_data/1 -> NR CRC Encoder/1
  Subsystem/1(end_out) -> valid_recover/3(end_in)
  Compare To Constant3/1 -> Logical Operator/2
  Logical Operator5/1 -> HDL Counter1/2, Switch1/2, Simple Dual Port RAM1/3  "wr_en"
  Compare To Constant5/1 -> Logical Operator6/1
  Data Type Conversion1/1 -> Simple Dual Port RAM1/1  "wr_din"
  HDL Counter4/1 -> Compare To Constant1/1, Compare To Constant4/1, Compare To Constant3/1, Compare To Constant2/1  "wr_addr"
  Compare To Constant6/1 -> Logical Operator6/2
  Constant2/1 -> Switch/3
  Compare To Constant2/1 -> HDL Counter5/2
  Compare To Constant1/1 -> Logical Operator/1
  NR CRC Encoder/2 -> Sample Control Bus Selector/1
  Sample Control Bus Creator/1 -> NR LDPC Encoder2/2
  Mux/1 -> ctrl_gen/1(data_in)
  Compare To Constant4/1 -> Logical Operator2/2
  Delay1/1 -> Mux/2
  Delay2/1 -> ctrl_gen/2(select_valid)
  process_valid/1 -> NR CRC Encoder/2
  ctrl_gen/1(data_out) -> bit_level_process/1  "INTERLEAVE"

== system tx2/Subsystem8/mapping_process_L1 ==
  data_in : Inport  OutDataTypeStr=boolean
  mapping_ctrl : Inport  Port=2  OutDataTypeStr=Bus: samplecontrol
  Constant : Constant  Value=sqrt(2)/2  OutDataTypeStr=fixdt(1,16,14)
  Constant1 : Constant  Value=-sqrt(2)/2  OutDataTypeStr=fixdt(1,16,14)
  Constant2 : Constant  Value=0  OutDataTypeStr=uint8
  Constant3 : Constant  Value=0  OutDataTypeStr=fixdt(1,16,14)
  Delay : Delay  DelayLength=1  InitialCondition=0  ShowEnablePort=on
      settings: InputPortMap=u0,e6
  Delay{1,5..8,10..12} (8 alike) : Delay  DelayLength=1  InitialCondition=0
  Delay{3..4,9,13} (4 alike) : Delay  InitialCondition=0
  Delay2 : Delay  DelayLength=1  InitialCondition=0  ShowEnablePort=on
      settings: InputPortMap=u0,e6
  Demux : Demux  Outputs=2
  Logical Operator : Logic  Operator=OR  AllPortsSameDT=off  OutDataTypeStr=boolean
  Logical Operator1 : Logic  AllPortsSameDT=off  OutDataTypeStr=boolean
  Logical Operator13 : Logic  Operator=NOT  AllPortsSameDT=off  OutDataTypeStr=boolean
  Real-Imag to Complex : RealImagToComplex
  Real-Imag to Complex1 : RealImagToComplex
  Sample Control Bus Creator : whdlutilities/Sample Control Bus Creator
      settings: SourceProductBaseCode=LH
  Sample Control Bus Creator1 : whdlutilities/Sample Control Bus Creator
      settings: SourceProductBaseCode=LH
  Sample Control Bus Selector : whdlutilities/Sample Control Bus Selector  OutputSignals=start,end,valid
      settings: SourceProductBaseCode=LH
  Switch{,1..3} (4 alike) : Switch  Criteria=u2 ~= 0  SaturateOnIntegerOverflow=off  InputSameDT=off
  "divide6 " : hdlsllib/Sources/HDL Counter  CountType=Count limited  CountInit=1  CountStep=1  CountMax=12  CountFromType=Initial value  CountFrom=1  CountResetPort=on  CountLoadPort=off  CountEnbPort=on  CountDirPort=off  CountHitOutputPort=on  CountDataType=Unsigned  CountWordLen=8  CountFracLen=0  CountSampTime=1
  divide6 1 : hdlsllib/Sources/HDL Counter  CountType=Count limited  CountInit=1  CountStep=1  CountMax=6*12  CountFromType=Initial value  CountFrom=1  CountResetPort=on  CountLoadPort=off  CountEnbPort=on  CountDirPort=off  CountHitOutputPort=off  CountDataType=Unsigned  CountWordLen=8  CountFracLen=0  CountSampTime=1
  data_out : Outport  VectorParamsAs1DForOutWhenUnconnected=off
      settings: SignalType=complex
  ctrl_mapping : Outport  Port=2  OutDataTypeStr=Bus: samplecontrol  VectorParamsAs1DForOutWhenUnconnected=off
  RB_ctrl : Outport  Port=3  OutDataTypeStr=Bus: samplecontrol  VectorParamsAs1DForOutWhenUnconnected=off
  RB_id : Outport  Port=4  OutDataTypeStr=uint8  VectorParamsAs1DForOutWhenUnconnected=off
  wires:
  Switch1/1 -> Real-Imag to Complex/2
  Switch/1 -> Real-Imag to Complex/1
  Delay/1 -> Demux/1
  Demux/1 -> Switch/2
  Demux/2 -> Switch1/2
  Real-Imag to Complex/1 -> Delay2/1
  Delay2/1 -> Delay6/1
  Delay3/1 -> Delay5/1
  Delay1/1 -> Delay2/2, Delay13/1
  mapping_ctrl/1 -> Sample Control Bus Selector/1
  "divide6 "/2 -> divide6 1/2, Delay11/1, Delay10/1  "count6"
  Logical Operator13/1 -> divide6 1/1, "divide6 "/1
  Sample Control Bus Selector/1 -> Delay9/1, Sample Control Bus Creator/1  "<start>"
  Sample Control Bus Selector/2 -> Sample Control Bus Creator/2  "<end>"
  Sample Control Bus Selector/3 -> Sample Control Bus Creator/3, Delay4/1, Delay1/1, Delay/2  "<valid>"
  Sample Control Bus Creator/1 -> Delay3/1
  divide6 1/1 -> Switch2/1  "RB_id"
  Delay4/1 -> Logical Operator13/1, "divide6 "/2, Delay12/1, Switch2/2, Logical Operator1/1
  Switch2/1 -> Delay7/1
  Constant2/1 -> Switch2/3
  Delay6/1 -> Switch3/1
  Logical Operator/1 -> Logical Operator1/2
  Delay9/1 -> Logical Operator/2
  Delay10/1 -> Logical Operator/1
  Logical Operator1/1 -> Delay8/1
  Delay8/1 -> Sample Control Bus Creator1/1
  Delay11/1 -> Sample Control Bus Creator1/2
  Delay12/1 -> Sample Control Bus Creator1/3
  Delay5/1 -> ctrl_mapping/1
  Delay7/1 -> RB_id/1
  Sample Control Bus Creator1/1 -> RB_ctrl/1
  data_in/1 -> Delay/1  "data_with_CP"
  Switch3/1 -> data_out/1
  Constant3/1 -> Real-Imag to Complex1/2, Real-Imag to Complex1/1
  Real-Imag to Complex1/1 -> Switch3/3
  Delay13/1 -> Switch3/2
  Constant/1 -> Switch1/3, Switch/3
  Constant1/1 -> Switch/1, Switch1/1

== system tx2/Subsystem9/BF ==
  layer_data_in1 : Inport
  BF_data_ctrl : Inport  Port=2  OutDataTypeStr=Bus: samplecontrol
  RB_id : Inport  Port=3  OutDataTypeStr=uint8
  RB_id_ctrl : Inport  Port=4  OutDataTypeStr=Bus: samplecontrol
  Delay{,3..8,10} (8 alike) : Delay  DelayLength=1  InitialCondition=0
  Delay1 : Delay  InitialCondition=0
  Delay2 : Delay  DelayLength=3  InitialCondition=0
  Delay9 : Delay  InitialCondition=0
  Logical Operator : Logic  Operator=NOT  AllPortsSameDT=off  OutDataTypeStr=boolean
  Mux : Mux  Inputs=8
  Product{,1..7} (8 alike) : Product  OutDataTypeStr=fixdt(1,16,14)  LockScale=on
  Sample Control Bus Selector : whdlutilities/Sample Control Bus Selector  OutputSignals=start,end,valid
      settings: SourceProductBaseCode=LH
  Sample Control Bus Selector1 : whdlutilities/Sample Control Bus Selector  OutputSignals=start,end,valid
      settings: SourceProductBaseCode=LH
  address controller : hdlsllib/Sources/HDL Counter  CountType=Count limited  CountInit=0  CountStep=1  CountMax=7  CountFromType=Initial value  CountFrom=0  CountResetPort=on  CountLoadPort=off  CountEnbPort=on  CountDirPort=off  CountHitOutputPort=off  CountDataType=Unsigned  CountWordLen=8  CountFracLen=0  CountSampTime=1
  rom_bf1 : Subsystem
  rom_bf2 : Subsystem
  rom_bf3 : Subsystem
  rom_bf4 : Subsystem
  rom_bf5 : Subsystem
  rom_bf6 : Subsystem
  rom_bf7 : Subsystem
  rom_bf8 : Subsystem
  process_bf : Outport  PortDimensions=8  VectorParamsAs1DForOutWhenUnconnected=off
  BF_ctrl : Outport  Port=2  OutDataTypeStr=Bus: samplecontrol  VectorParamsAs1DForOutWhenUnconnected=off
  RB_n_bf : Outport  Port=3  VectorParamsAs1DForOutWhenUnconnected=off
  wires:
  Delay1/1 -> Product7/1, Product6/1, Product5/1, Product4/1, Product3/1, Product2/1, Product1/1, Product/1
  rom_bf1/1(data_out) -> Product/2
  Product/1 -> Delay/1
  Delay2/1 -> BF_ctrl/1  "BF_ctrl"
  address controller/1 -> rom_bf7/1(address), rom_bf8/1(address), rom_bf6/1(address), rom_bf5/1(address), rom_bf4/1(address), rom_bf3/1(address), rom_bf2/1(address), rom_bf1/1(address)
  Delay9/1 -> RB_n_bf/1  "RB_ID"
  RB_id_ctrl/1 -> Sample Control Bus Selector1/1
  BF_data_ctrl/1 -> Delay2/1, Sample Control Bus Selector/1
  Sample Control Bus Selector1/2 -> address controller/2  "<end>"
  RB_id/1 -> Delay9/1
  layer_data_in1/1 -> Delay1/1
  Sample Control Bus Selector/3 -> rom_bf2/2(read_en), rom_bf1/2(read_en), rom_bf3/2(read_en), rom_bf4/2(read_en), rom_bf5/2(read_en), rom_bf6/2(read_en), rom_bf7/2(read_en), rom_bf8/2(read_en)  "<valid>"
  Product1/1 -> Delay3/1
  Product2/1 -> Delay4/1
  Product4/1 -> Delay6/1
  Product3/1 -> Delay5/1
  Product5/1 -> Delay7/1
  Product6/1 -> Delay8/1
  rom_bf2/1(data_out) -> Product1/2
  rom_bf3/1(data_out) -> Product2/2
  rom_bf4/1(data_out) -> Product3/2
  rom_bf5/1(data_out) -> Product4/2
  rom_bf6/1(data_out) -> Product5/2
  Product7/1 -> Delay10/1
  rom_bf7/1(data_out) -> Product6/2
  rom_bf8/1(data_out) -> Product7/2
  Delay3/1 -> Mux/2
  Delay4/1 -> Mux/3
  Delay5/1 -> Mux/4
  Delay10/1 -> Mux/8
  Delay8/1 -> Mux/7
  Delay7/1 -> Mux/6
  Delay6/1 -> Mux/5
  Delay/1 -> Mux/1
  Mux/1 -> process_bf/1
  Sample Control Bus Selector1/3 -> Logical Operator/1  "<valid>"
  Logical Operator/1 -> address controller/1

== system tx2/Subsystem9/OFDM_process1 ==
  process_bf : Inport
  BF_ctrl : Inport  Port=2
  Demux : Demux  Outputs=8
  OFDM_process1_bf1 : Subsystem
  OFDM_process1_bf2 : Subsystem
  OFDM_process1_bf3 : Subsystem
  OFDM_process1_bf4 : Subsystem
  OFDM_process1_bf5 : Subsystem
  OFDM_process1_bf6 : Subsystem
  OFDM_process1_bf7 : Subsystem
  OFDM_process1_bf8 : Subsystem
  OFDM_bf1 : Outport
  OFDM_ctrl_bf1 : Outport  Port=2
  OFDM_bf2 : Outport  Port=3
  OFDM_ctrl_bf2 : Outport  Port=4
  OFDM_bf3 : Outport  Port=5
  OFDM_ctrl_bf3 : Outport  Port=6
  OFDM_bf4 : Outport  Port=7
  OFDM_ctrl_bf4 : Outport  Port=8
  OFDM_bf5 : Outport  Port=9
  OFDM_ctrl_bf5 : Outport  Port=10
  OFDM_bf6 : Outport  Port=11
  OFDM_ctrl_bf6 : Outport  Port=12
  OFDM_bf7 : Outport  Port=13
  OFDM_ctrl_bf7 : Outport  Port=14
  OFDM_bf8 : Outport  Port=15
  OFDM_ctrl_bf8 : Outport  Port=16
  wires:
  Demux/3 -> OFDM_process1_bf3/1(data)  "bf3"
  Demux/1 -> OFDM_process1_bf1/1(data)  "bf1"
  BF_ctrl/1 -> OFDM_process1_bf7/2(BF_ctrl), OFDM_process1_bf8/2(BF_ctrl), OFDM_process1_bf6/2(BF_ctrl), OFDM_process1_bf5/2(BF_ctrl), OFDM_process1_bf4/2(BF_ctrl), OFDM_process1_bf3/2(BF_ctrl), OFDM_process1_bf2/2(BF_ctrl), OFDM_process1_bf1/2(BF_ctrl)
  Demux/5 -> OFDM_process1_bf5/1(data)  "bf5"
  OFDM_process1_bf1/2(OFDM_ctrl_process) -> OFDM_ctrl_bf1/1
  OFDM_process1_bf2/2(OFDM_ctrl_process) -> OFDM_ctrl_bf2/1
  Demux/2 -> OFDM_process1_bf2/1(data)  "bf2"
  Demux/4 -> OFDM_process1_bf4/1(data)  "bf4"
  OFDM_process1_bf8/2(OFDM_ctrl_process) -> OFDM_ctrl_bf8/1
  Demux/8 -> OFDM_process1_bf8/1(data)  "bf8"
  Demux/7 -> OFDM_process1_bf7/1(data)  "bf7"
  Demux/6 -> OFDM_process1_bf6/1(data)  "bf6"
  OFDM_process1_bf7/2(OFDM_ctrl_process) -> OFDM_ctrl_bf7/1
  OFDM_process1_bf6/1(OFDM_process) -> OFDM_bf6/1
  OFDM_process1_bf3/1(OFDM_process) -> OFDM_bf3/1
  OFDM_process1_bf6/2(OFDM_ctrl_process) -> OFDM_ctrl_bf6/1
  OFDM_process1_bf5/1(OFDM_process) -> OFDM_bf5/1
  OFDM_process1_bf1/1(OFDM_process) -> OFDM_bf1/1
  OFDM_process1_bf8/1(OFDM_process) -> OFDM_bf8/1
  OFDM_process1_bf4/2(OFDM_ctrl_process) -> OFDM_ctrl_bf4/1
  OFDM_process1_bf3/2(OFDM_ctrl_process) -> OFDM_ctrl_bf3/1
  OFDM_process1_bf5/2(OFDM_ctrl_process) -> OFDM_ctrl_bf5/1
  process_bf/1 -> Demux/1
  OFDM_process1_bf7/1(OFDM_process) -> OFDM_bf7/1
  OFDM_process1_bf4/1(OFDM_process) -> OFDM_bf4/1
  OFDM_process1_bf2/1(OFDM_process) -> OFDM_bf2/1
